simulink model "platoon_project_string_stability"  (Simulink 8.9)
settings: Solver=VariableStepAuto  StartTime=0.0  StopTime=12  FixedStep=0.1  RelTol=1e-3  EnableMultiTasking=on
values from neighbouring files (symbols this model uses):
  k1 = 1.3244    [platoon_stability.m]    (also in platoon_stability_ed.m = 0.0244)
  k2 = -1.2211    [platoon_stability.m]    (also in platoon_stability_ed.m = -1.7211)
  q = 0.1    [platoon_stability.m]    (also in platoon_stability_ed.m = 0.2)
  tau = 1.34    [platoon_stability.m]    (also in platoon_stability_ed.m = 1.24)
  tnet_table = [57.5127074443 119.897368421 182.282029398 223.675296349 261.549751738 274.206057597 279.305263158 283.689473684 288.073684211 292.467532318 296.875779086 301.284025854 ... (400 elements, 20x20)]    [enginemap.mat]    (also in genmap.m = griddata(map_ford(:,1), map_ford(:,4), map_ford(:,2), we_tab)
  we_max = 471.2    [enginemap.mat]    (also in genmap.m = max(map_ford(:,1)))
  we_min = 57.6    [enginemap.mat]    (also in genmap.m = min(map_ford(:,1)))
undefined symbols (not defined in the file or in its folder): c_aero, delay_brake, F_roll, h, I_e, I_wheel, KB, mass, max_throttle, max_throttle_rate, min_throttle, mu_B, mu_C, mu_D, mu_E, P_po, Rdrive, sigbuilder_block, tau_brake, tau_throttle, throttle_o, w_wheel_o, we_o, x_dot_o
libraries: simulink x8
(part 3 of 3)

== matlab function                ACC Based On DIstance             ==
  data: ei input double; Throttle_Angle_err output double; Pmc_err output double
function [Throttle_Angle_err,Pmc_err] = acc(ei)

if ei > 0
    Throttle_Angle_err =  1;
    Pmc_err = 0;
else 
    Throttle_Angle_err =  0;
    Pmc_err =  1; 
end

end

== matlab function                ACC Based On DIstance            ==
  data: ei input double; Throttle_Angle_err output double; Pmc_err output double
function [Throttle_Angle_err,Pmc_err] = acc(ei)

if ei > 0
    Throttle_Angle_err =  1;
    Pmc_err = 0;
else 
    Throttle_Angle_err =  0;
    Pmc_err =  1; 
end

end

== matlab function                ACC Based On DIstance               ==
  data: ei input double; Throttle_Angle_err output double; Pmc_err output double
function [Throttle_Angle_err,Pmc_err] = acc(ei)

if ei > 0
    Throttle_Angle_err =  1;
    Pmc_err = 0;
else 
    Throttle_Angle_err =  0;
    Pmc_err =  1; 
end

end

== matlab function                ACC Based On DIstance              ==
  data: ei input double; Throttle_Angle_err output double; Pmc_err output double
function [Throttle_Angle_err,Pmc_err] = acc(ei)

if ei > 0
    Throttle_Angle_err =  1;
    Pmc_err = 0;
else 
    Throttle_Angle_err =  0;
    Pmc_err =  1; 
end

end
